simulink model "balacingRobotControl"  (R2020b)
settings: Solver=VariableStepAuto  StartTime=0.0  StopTime=12  RelTol=1e-3
values from neighbouring files (symbols this model uses):
  drv =     [parameters.mat]
  Fv1 = [Fv1_11,Fv1_12;Fv1_21,Fv1_22]    [LAB4.m]
  gbox =     [parameters.mat]
  M11 = 2*wheel.Iyy+2*(gbox.N^2)*mot.rot.Iyy+(body.m+2*wheel.m+2*mot.rot.m)*(wheel.r^2)    [LAB4.m]
  M22 = body.Iyy+2*((1-gbox.N)^(2))*mot.rot.Iyy+body.m*(body.zb^2)+2*mot.rot.m*(mot.rot.zb)^2    [LAB4.m]
  ms22g = 1/g    (= 0.101936799185)    [DataLAB4.m]    (also in parameters.mat)
  sens =     [parameters.mat]
  Ts = 1e-2    (= 0.01)    [DataLAB4.m]    (also in parameters.mat)
  ua2tau = 2*gbox.N*mot.R*[1;-1]    [LAB4.m]
  wheel =     [parameters.mat]
undefined symbols (not defined in the file or in its folder): DiscIntNeverNeededParam, K, N_u, N_x
settings Model: Creator=Alessandro  LastModifiedBy=mioma
settings DebuggingCC: UnconnectedInputMsg=none  UnconnectedOutputMsg=none  UnconnectedLineMsg=none  SFMachineParentedDataDiag=error
settings SimscapeCC: SimscapeLogType=all  SimscapeLogLimitData=off

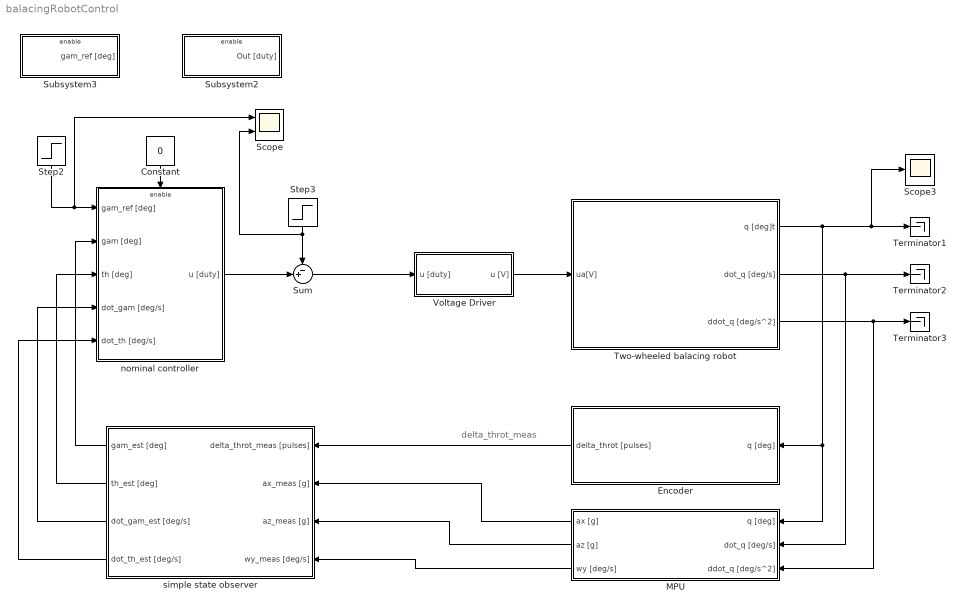
== system balacingRobotControl ==
  note: delta_throt_meas
  Constant : Constant  Value=0
  Encoder : Subsystem
  MPU : Subsystem
  Scope : Scope  NumInputPorts=2
  Scope3 : Scope
  Step2 : Step  Time=0  After=(0.1/wheel.r)*rad2deg*1  SampleTime=Ts
  Step3 : Step  Time=10  After=5.0/drv.duty2V  SampleTime=Ts
  Subsystem2 : Subsystem
  Subsystem3 : Subsystem
  Sum : Sum  Inputs=-+|
  Terminator1 : Terminator
  Terminator2 : Terminator
  Terminator3 : Terminator
  Two-wheeled balacing robot : Subsystem
  Voltage Driver : Subsystem
  nominal controller : Subsystem
  simple state observer : Subsystem
  wires:
  Two-wheeled balacing robot/3(ddot_q [deg/s^2]) -> Terminator3/1, MPU/3(ddot_q [deg/s^2])
  MPU/1(ax [g]) -> simple state observer/2(ax_meas [g])
  Step3/1 -> Scope/2, Sum/1
  MPU/3(wy [deg/s]) -> simple state observer/4(wy_meas [deg/s])
  simple state observer/2(th_est [deg]) -> nominal controller/3(th [deg])
  Encoder/1(delta_throt [pulses]) -> simple state observer/1(delta_throt_meas [pulses])
  MPU/2(az [g]) -> simple state observer/3(az_meas [g])
  Sum/1 -> Voltage Driver/1(u [duty])
  simple state observer/1(gam_est [deg]) -> nominal controller/2(gam [deg])
  Two-wheeled balacing robot/1(q [deg]t) -> Scope3/1, Terminator1/1, MPU/1(q [deg]), Encoder/1(q [deg])
  Voltage Driver/1(u [V]) -> Two-wheeled balacing robot/1(ua[V])
  nominal controller/1(u [duty]) -> Sum/2
  simple state observer/4(dot_th_est [deg/s]) -> nominal controller/5(dot_th [deg/s])
  Two-wheeled balacing robot/2(dot_q [deg/s]) -> Terminator2/1, MPU/2(dot_q [deg/s])
  simple state observer/3(dot_gam_est [deg/s]) -> nominal controller/4(dot_gam [deg/s])
  Constant/1 -> nominal controller/Enable
  Step2/1 -> Scope/1, nominal controller/1(gam_ref [deg])

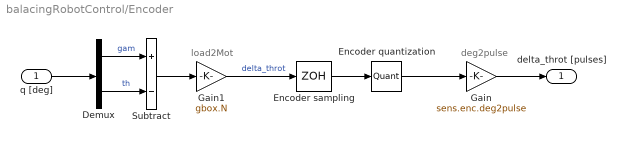
== system balacingRobotControl/Encoder ==
  note: load2Mot
  note: deg2pulse
  q [deg] : Inport
  Demux : Demux  Outputs=2
  Encoder quantization : Quantizer  QuantizationInterval=sens.enc.pulse2deg
  Encoder sampling : ZeroOrderHold  SampleTime=Ts
  Gain : Gain  Gain=sens.enc.deg2pulse
  Gain1 : Gain  Gain=gbox.N
  Subtract : Sum  Inputs=+-
  delta_throt [pulses] : Outport
  wires:
  Gain1/1 -> Encoder sampling/1  "delta_throt"
  Demux/1 -> Subtract/1  "gam"
  Gain/1 -> delta_throt [pulses]/1
  Subtract/1 -> Gain1/1
  Demux/2 -> Subtract/2  "th"
  q [deg]/1 -> Demux/1
  Encoder quantization/1 -> Gain/1
  Encoder sampling/1 -> Encoder quantization/1

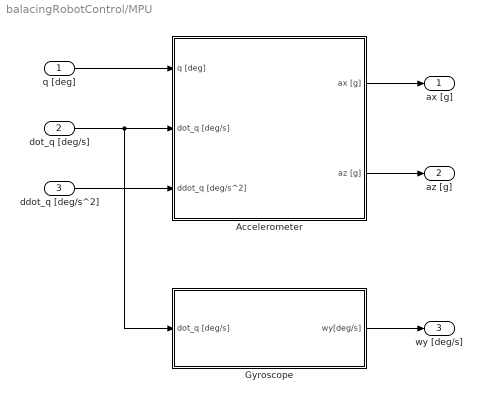
== system balacingRobotControl/MPU ==
  q [deg] : Inport
  dot_q [deg/s] : Inport  Port=2
  ddot_q [deg/s^2] : Inport  Port=3
  Accelerometer : Subsystem
  Gyroscope : Subsystem
  ax [g] : Outport
  az [g] : Outport  Port=2
  wy [deg/s] : Outport  Port=3
  wires:
  Gyroscope/1(wy[deg/s]) -> wy [deg/s]/1
  q [deg]/1 -> Accelerometer/1(q [deg])
  dot_q [deg/s]/1 -> Gyroscope/1(dot_q [deg/s]), Accelerometer/2(dot_q [deg/s])
  ddot_q [deg/s^2]/1 -> Accelerometer/3(ddot_q [deg/s^2])
  Accelerometer/2(az [g]) -> az [g]/1
  Accelerometer/1(ax [g]) -> ax [g]/1

== system balacingRobotControl/Subsystem2 ==
  Enable : EnablePort
  Constant : Constant  Value=5.0/drv.duty2V
  Out [duty] : Outport
  wires:
  Constant/1 -> Out [duty]/1

== system balacingRobotControl/Subsystem3 ==
  Enable : EnablePort
  Constant : Constant  Value=(0.1/wheel.r)*rad2deg
  gam_ref [deg] : Outport
  wires:
  Constant/1 -> gam_ref [deg]/1

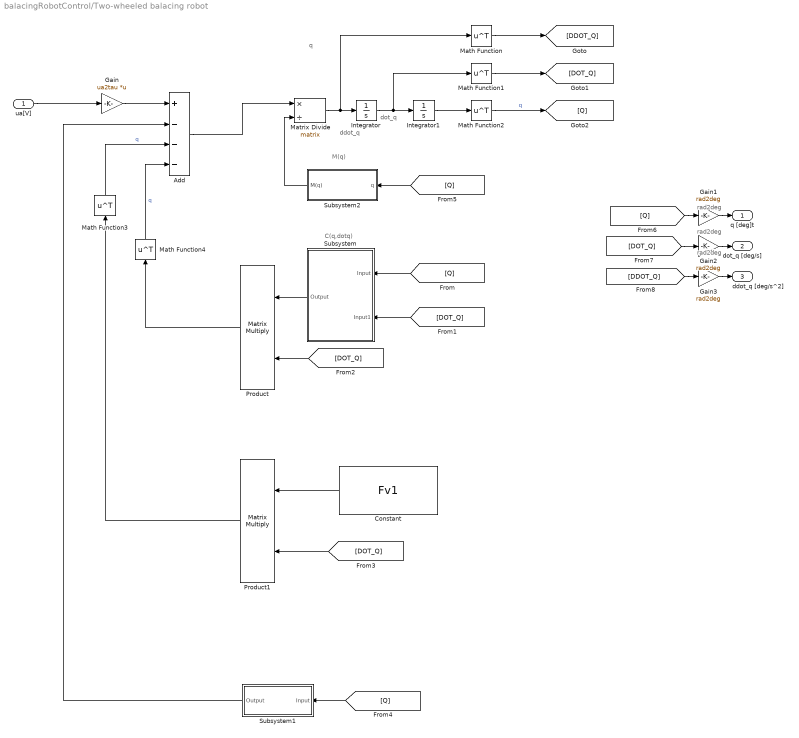
== system balacingRobotControl/Two-wheeled balacing robot ==
  note: rad2deg
  note: C(q,dotq)
  note: M(q)
  note: dot_q
  note: q
  note: ddot_q
  note: rad2deg
  note: rad2deg
  ua[V] : Inport
  Add : Sum  Inputs=+---
  Constant : Constant  Value=Fv1
  Gain : Gain  Gain=ua2tau  Multiplication=Matrix(K*u)
  Gain1 : Gain  Gain=rad2deg
  Gain2 : Gain  Gain=rad2deg
  Gain3 : Gain  Gain=rad2deg
  Integrator : Integrator
  Integrator1 : Integrator
  Math Function{,1..4} (5 alike) : Math  Operator=transpose  SaturateOnIntegerOverflow=on
  Matrix Divide : Product  Inputs=*/  Multiplication=Matrix(*)
  Product : Product  Multiplication=Matrix(*)
  Product1 : Product  Multiplication=Matrix(*)
  Subsystem : Subsystem
  Subsystem1 : Subsystem
  Subsystem2 : Subsystem
  q [deg]t : Outport
  dot_q [deg/s] : Outport  Port=2
  ddot_q [deg/s^2] : Outport  Port=3
  wires:
  Integrator1/1 -> Math Function2/1
  [DDOT_Q] -> Gain3/1
  [DOT_Q] -> Gain2/1
  Gain2/1 -> dot_q [deg/s]/1
  Matrix Divide/1 -> Math Function/1, Integrator/1
  [DOT_Q] -> Subsystem/2(Input1)
  [Q] -> Subsystem2/1(q)
  Subsystem/1(Output) -> Product/1
  [DOT_Q] -> Product1/2
  Constant/1 -> Product1/1
  [Q] -> Subsystem/1(Input)
  Integrator/1 -> Math Function1/1, Integrator1/1
  ua[V]/1 -> Gain/1
  [Q] -> Subsystem1/1(Input)
  [Q] -> Gain1/1
  Gain1/1 -> q [deg]t/1
  [DOT_Q] -> Product/2
  Gain3/1 -> ddot_q [deg/s^2]/1
  Math Function/1 -> [DDOT_Q]
  Math Function1/1 -> [DOT_Q]
  Math Function2/1 -> [Q]  "q"
  Gain/1 -> Add/1
  Product1/1 -> Math Function3/1
  Product/1 -> Math Function4/1
  Subsystem1/1(Output) -> Add/2
  Math Function3/1 -> Add/3  "q"
  Math Function4/1 -> Add/4  "q"
  Add/1 -> Matrix Divide/1
  Subsystem2/1(M(q)) -> Matrix Divide/2

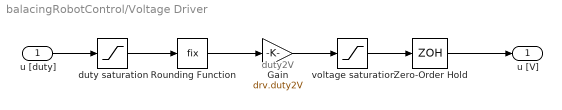
== system balacingRobotControl/Voltage Driver ==
  note: duty2V
  u [duty] : Inport
  Gain : Gain  Gain=drv.duty2V
  Rounding Function : Rounding  Operator=fix
  Zero-Order Hold : ZeroOrderHold  SampleTime=Ts
  duty saturation : Saturate  UpperLimit=drv.dutymax  LowerLimit=-drv.dutymax
  voltage saturation : Saturate  UpperLimit=drv.Vbus  LowerLimit=-drv.Vbus
  u [V] : Outport
  wires:
  Zero-Order Hold/1 -> u [V]/1
  voltage saturation/1 -> Zero-Order Hold/1
  duty saturation/1 -> Rounding Function/1
  u [duty]/1 -> duty saturation/1
  Gain/1 -> voltage saturation/1
  Rounding Function/1 -> Gain/1

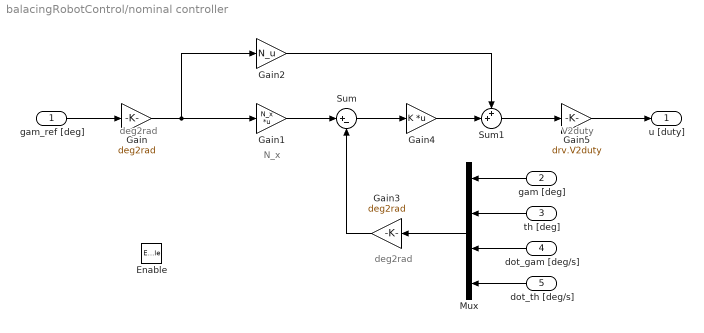
== system balacingRobotControl/nominal controller ==
  note: N_x
  note: deg2rad
  note: deg2rad
  note: V2duty
  gam_ref [deg] : Inport
  gam [deg] : Inport  Port=2
  th [deg] : Inport  Port=3
  dot_gam [deg/s] : Inport  Port=4
  dot_th [deg/s] : Inport  Port=5
  Enable : EnablePort
  Gain : Gain  Gain=deg2rad
  Gain1 : Gain  Gain=N_x  Multiplication=Matrix(K*u)
  Gain2 : Gain  Gain=N_u
  Gain3 : Gain  Gain=deg2rad
  Gain4 : Gain  Gain=K  Multiplication=Matrix(K*u)
  Gain5 : Gain  Gain=drv.V2duty
  Mux : Mux
  Sum : Sum  Inputs=|+-
  Sum1 : Sum  Inputs=++|
  u [duty] : Outport
  wires:
  dot_th [deg/s]/1 -> Mux/4
  Sum1/1 -> Gain5/1
  gam_ref [deg]/1 -> Gain/1
  th [deg]/1 -> Mux/2
  Gain3/1 -> Sum/2
  Gain2/1 -> Sum1/1
  Mux/1 -> Gain3/1
  Gain1/1 -> Sum/1
  Gain5/1 -> u [duty]/1
  dot_gam [deg/s]/1 -> Mux/3
  Gain4/1 -> Sum1/2
  Sum/1 -> Gain4/1
  gam [deg]/1 -> Mux/1
  Gain/1 -> Gain2/1, Gain1/1

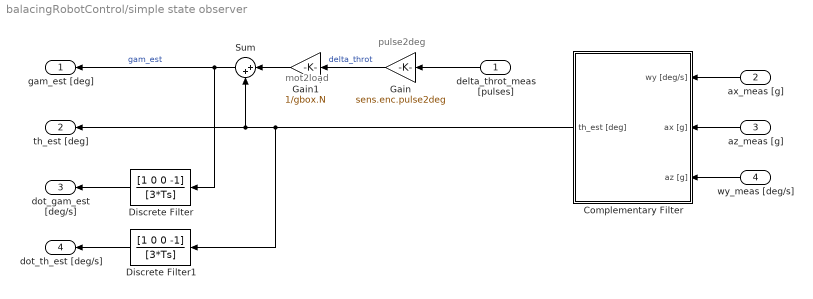
== system balacingRobotControl/simple state observer ==
  note: mot2load
  note: pulse2deg
  delta_throt_meas [pulses] : Inport
  ax_meas [g] : Inport  Port=2
  az_meas [g] : Inport  Port=3
  wy_meas [deg/s] : Inport  Port=4
  Complementary Filter : Subsystem
  Discrete Filter : DiscreteFilter  Numerator=[1 0 0 -1]  Denominator=[3*Ts]  SampleTime=Ts
  Discrete Filter1 : DiscreteFilter  Numerator=[1 0 0 -1]  Denominator=[3*Ts]  SampleTime=Ts
  Gain : Gain  Gain=sens.enc.pulse2deg
  Gain1 : Gain  Gain=1/gbox.N
  Sum : Sum  Inputs=|++
  gam_est [deg] : Outport
  th_est [deg] : Outport  Port=2
  dot_gam_est [deg/s] : Outport  Port=3
  dot_th_est [deg/s] : Outport  Port=4
  wires:
  Discrete Filter/1 -> dot_gam_est [deg/s]/1
  Gain1/1 -> Sum/1
  Discrete Filter1/1 -> dot_th_est [deg/s]/1
  Complementary Filter/1(th_est [deg]) -> Discrete Filter1/1, Sum/2, th_est [deg]/1
  Gain/1 -> Gain1/1  "delta_throt"
  Sum/1 -> Discrete Filter/1, gam_est [deg]/1  "gam_est"
  ax_meas [g]/1 -> Complementary Filter/1(wy [deg/s])
  delta_throt_meas [pulses]/1 -> Gain/1
  wy_meas [deg/s]/1 -> Complementary Filter/3(az [g])
  az_meas [g]/1 -> Complementary Filter/2(ax [g])

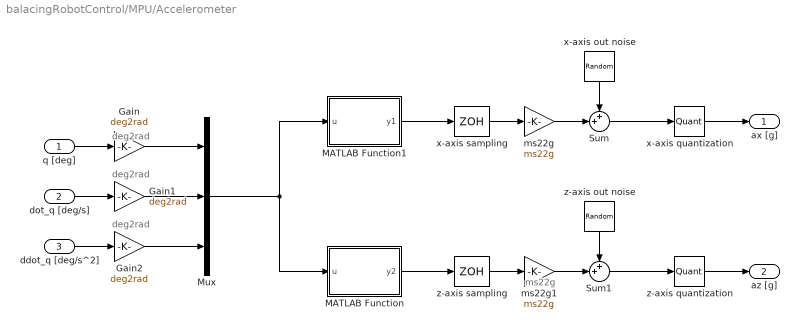
== system balacingRobotControl/MPU/Accelerometer ==
  note: ms22g
  note: deg2rad
  note: deg2rad
  note: deg2rad
  q [deg] : Inport
  dot_q [deg/s] : Inport  Port=2
  ddot_q [deg/s^2] : Inport  Port=3
  Gain : Gain  Gain=deg2rad
  Gain1 : Gain  Gain=deg2rad
  Gain2 : Gain  Gain=deg2rad
  MATLAB Function : MATLAB Function  TreatAsAtomicUnit=on
  MATLAB Function1 : MATLAB Function  TreatAsAtomicUnit=on
  Mux : Mux  Inputs=3
  Sum : Sum  Inputs=++|
  Sum1 : Sum  Inputs=++|
  ms22g : Gain  Gain=ms22g
  ms22g1 : Gain  Gain=ms22g
  x-axis out noise : RandomNumber  Variance=sens.mpu.acc.noisevar  SampleTime=Ts
  x-axis quantization : Quantizer  QuantizationInterval=sens.mpu.acc.LSB2g
  x-axis sampling : ZeroOrderHold  SampleTime=Ts
  z-axis out noise : RandomNumber  Variance=sens.mpu.acc.noisevar  SampleTime=Ts
  z-axis quantization : Quantizer  QuantizationInterval=sens.mpu.acc.LSB2g
  z-axis sampling : ZeroOrderHold  SampleTime=Ts
  ax [g] : Outport
  az [g] : Outport  Port=2
  wires:
  q [deg]/1 -> Gain/1
  Gain/1 -> Mux/1
  dot_q [deg/s]/1 -> Gain1/1
  Gain1/1 -> Mux/2
  Gain2/1 -> Mux/3
  ddot_q [deg/s^2]/1 -> Gain2/1
  x-axis quantization/1 -> ax [g]/1
  x-axis out noise/1 -> Sum/1
  Sum/1 -> x-axis quantization/1
  ms22g/1 -> Sum/2
  x-axis sampling/1 -> ms22g/1
  z-axis quantization/1 -> az [g]/1
  z-axis sampling/1 -> ms22g1/1
  Sum1/1 -> z-axis quantization/1
  z-axis out noise/1 -> Sum1/1
  ms22g1/1 -> Sum1/2
  Mux/1 -> MATLAB Function1/1(u), MATLAB Function/1(u)
  MATLAB Function/1(y2) -> z-axis sampling/1
  MATLAB Function1/1(y1) -> x-axis sampling/1

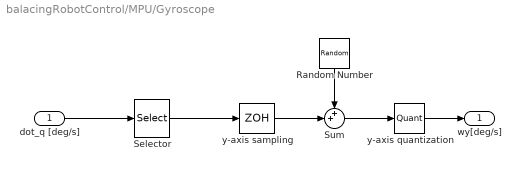
== system balacingRobotControl/MPU/Gyroscope ==
  dot_q [deg/s] : Inport
  Random Number : RandomNumber  Variance=sens.mpu.gyro.noisevar  SampleTime=Ts
  Selector : Selector  InputPortWidth=2  IndexOptions=Index vector (dialog)  Indices=2  OutputSizes=1
  Sum : Sum  Inputs=++|
  y-axis quantization : Quantizer  QuantizationInterval=sens.mpu.gyro.LSB2degs
  y-axis sampling : ZeroOrderHold  SampleTime=Ts
  wy[deg/s] : Outport
  wires:
  dot_q [deg/s]/1 -> Selector/1
  y-axis quantization/1 -> wy[deg/s]/1
  Sum/1 -> y-axis quantization/1
  Random Number/1 -> Sum/1
  y-axis sampling/1 -> Sum/2
  Selector/1 -> y-axis sampling/1

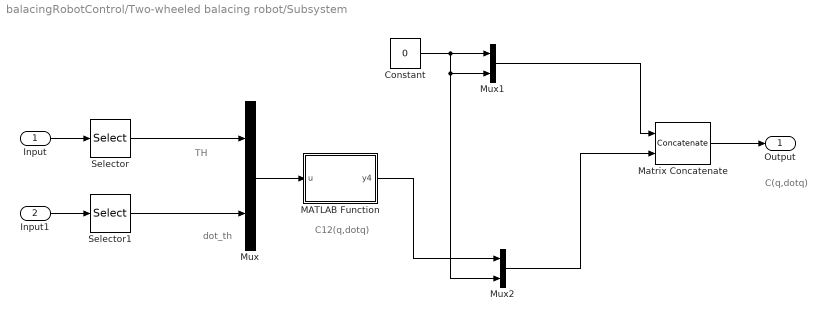
== system balacingRobotControl/Two-wheeled balacing robot/Subsystem ==
  note: dot_th
  note: TH
  note: C12(q,dotq)
  note: C(q,dotq)
  Input : Inport
  Input1 : Inport  Port=2
  Constant : Constant  Value=0
  MATLAB Function : MATLAB Function  TreatAsAtomicUnit=on
  Matrix Concatenate : Concatenate  Mode=Multidimensional array  ConcatenateDimension=2
  Mux : Mux  Inputs=2
  Mux1 : Mux  Inputs=2
  Mux2 : Mux  Inputs=2
  Selector : Selector  IndexMode=Zero-based  InputPortWidth=2  IndexOptions=Index vector (dialog)  Indices=1  OutputSizes=1
  Selector1 : Selector  IndexMode=Zero-based  InputPortWidth=2  IndexOptions=Index vector (dialog)  Indices=1  OutputSizes=1
  Output : Outport
  wires:
  Input/1 -> Selector/1
  Selector/1 -> Mux/1
  Constant/1 -> Mux2/2, Mux1/2, Mux1/1
  Input1/1 -> Selector1/1
  Mux2/1 -> Matrix Concatenate/2
  Mux1/1 -> Matrix Concatenate/1
  Selector1/1 -> Mux/2
  Matrix Concatenate/1 -> Output/1
  Mux/1 -> MATLAB Function/1(u)
  MATLAB Function/1(y4) -> Mux2/1

== system balacingRobotControl/Two-wheeled balacing robot/Subsystem1 ==
  note: q
  Input : Inport
  Constant : Constant  Value=0
  MATLAB Function : MATLAB Function  TreatAsAtomicUnit=on
  Mux : Mux  Inputs=2
  Selector : Selector  IndexMode=Zero-based  InputPortWidth=2  IndexOptions=Index vector (dialog)  Indices=1  OutputSizes=1
  Output : Outport
  wires:
  Input/1 -> Selector/1
  Constant/1 -> Mux/1
  Mux/1 -> Output/1
  MATLAB Function/1(y3) -> Mux/2
  Selector/1 -> MATLAB Function/1(u)

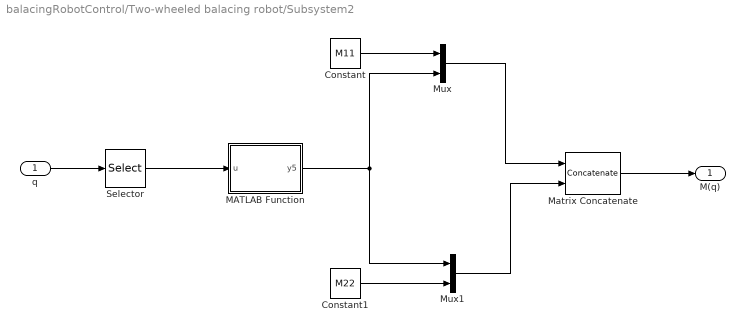
== system balacingRobotControl/Two-wheeled balacing robot/Subsystem2 ==
  q : Inport
  Constant : Constant  Value=M11
  Constant1 : Constant  Value=M22
  MATLAB Function : MATLAB Function  TreatAsAtomicUnit=on
  Matrix Concatenate : Concatenate  Mode=Multidimensional array  ConcatenateDimension=2
  Mux : Mux  Inputs=2
  Mux1 : Mux  Inputs=2
  Selector : Selector  IndexMode=Zero-based  InputPortWidth=2  IndexOptions=Index vector (dialog)  Indices=1  OutputSizes=1
  M(q) : Outport
  wires:
  Mux/1 -> Matrix Concatenate/1
  Matrix Concatenate/1 -> M(q)/1
  Mux1/1 -> Matrix Concatenate/2
  Constant1/1 -> Mux1/2
  Constant/1 -> Mux/1
  q/1 -> Selector/1
  Selector/1 -> MATLAB Function/1(u)
  MATLAB Function/1(y5) -> Mux1/1, Mux/2

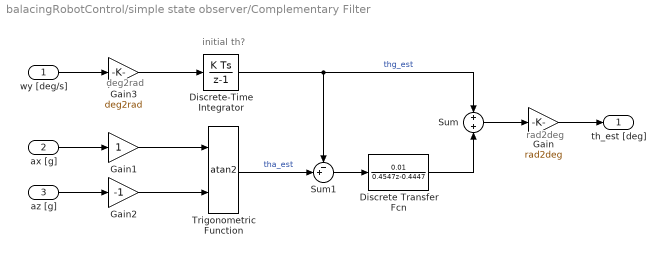
== system balacingRobotControl/simple state observer/Complementary Filter ==
  note: initial th?
  note: rad2deg
  note: deg2rad
  wy [deg/s] : Inport
  ax [g] : Inport  Port=2
  az [g] : Inport  Port=3
  Discrete Transfer Fcn : DiscreteTransferFcn  Numerator=[0.01]  Denominator=[0.4547 -0.4447]  SampleTime=Ts
  Discrete-Time Integrator : DiscreteIntegrator  SampleTime=Ts  ICPrevOutput=DiscIntNeverNeededParam  ICPrevScaledInput=DiscIntNeverNeededParam
  Gain : Gain  Gain=rad2deg
  Gain1 : Gain
  Gain2 : Gain  Gain=-1
  Gain3 : Gain  Gain=deg2rad
  Sum : Sum  Inputs=+|+
  Sum1 : Sum  Inputs=-+|
  Trigonometric Function : Trigonometry  Operator=atan2
  th_est [deg] : Outport
  wires:
  Gain/1 -> th_est [deg]/1
  Sum/1 -> Gain/1
  ax [g]/1 -> Gain1/1
  Gain1/1 -> Trigonometric Function/1
  az [g]/1 -> Gain2/1
  Gain2/1 -> Trigonometric Function/2
  wy [deg/s]/1 -> Gain3/1
  Gain3/1 -> Discrete-Time Integrator/1
  Trigonometric Function/1 -> Sum1/2  "tha_est"
  Discrete-Time Integrator/1 -> Sum/1, Sum1/1  "thg_est"
  Sum1/1 -> Discrete Transfer Fcn/1
  Discrete Transfer Fcn/1 -> Sum/2

== matlab function balacingRobotControl/MPU/Accelerometer/MATLAB Function ==
  data: u input; y2 output
function y2 = zaxis(u)
wheel.r=0.034;
sens.mpu.zb=0.0135;
g=9.81;
y2 = wheel.r*u(5)*sin(u(2)) - sens.mpu.zb*(u(4))^2 - g*cos(u(2));

== matlab function balacingRobotControl/Two-wheeled balacing robot/Subsystem1/MATLAB Function ==
  data: u input; y3 output
function y3 = gf(u)
body.m=1.0555;
body.zb=0.046047844623401;
mot.rot.m=0.07525;
mot.rot.zb=-0.007;
g=9.81;
g2=-(body.m*body.zb+2*mot.rot.m*mot.rot.zb)*g;
y3=g2*sin(u);

== matlab function balacingRobotControl/Two-wheeled balacing robot/Subsystem/MATLAB Function ==
  data: u input; y4 output
function y4 = dfcn(u)
body.m=1.0555;
body.zb=0.046047844623401;
mot.rot.m=0.07525;
mot.rot.zb=-0.007;
wheel.r=0.034;
C12=(body.m*body.zb+2*mot.rot.m*mot.rot.zb)*wheel.r;
y4=-C12*sin(u(1))*u(2);

== matlab function balacingRobotControl/Two-wheeled balacing robot/Subsystem2/MATLAB Function ==
  data: u input; y5 output
function y5 = fcn(u)
gbox.N=30;
mot.rot.Iyy=8.807636250000001e-06;
body.m=1.0555;
body.zb=0.046047844623401;
mot.rot.m=0.07525;
mot.rot.zb=-0.007;
wheel.r=0.034000000000000;
x=2*gbox.N*(1-gbox.N)*mot.rot.Iyy;
y5 = x + (body.m*body.zb+2*mot.rot.m*mot.rot.zb)*wheel.r*cos(u);

== matlab function balacingRobotControl/MPU/Accelerometer/MATLAB Function1 ==
  data: u input; y1 output
function y1 = xaxis(u)
sens.mpu.zb=0.0135;
wheel.r=0.034;
g=9.81;
y1 = wheel.r*u(5)*cos(u(2)) + sens.mpu.zb*u(6) + g*sin(u(2));
